simulink model "TrainSimulation_trial"  (R2021a)
settings: Solver=VariableStepAuto  StartTime=0.0  StopTime=10.0  MaxStep=0.01  RelTol=1e-3
values from neighbouring files (symbols this model uses):
  g = 9.8    [TrainSimulation_run.m]
  k = 20    [MassSpringDamper_run.m]    (also in PID_SpringDamper_run.m; PID_block_run.m; TrainSimulation_run.m = 1; TransferFunctionModel_run.m)
  M1 = 1    [TrainSimulation_run.m]
  M2 = 0.5    [TrainSimulation_run.m]
  mu = 0.02    [TrainSimulation_run.m]
settings Model: Creator=shinyh  LastModifiedBy=shinyh

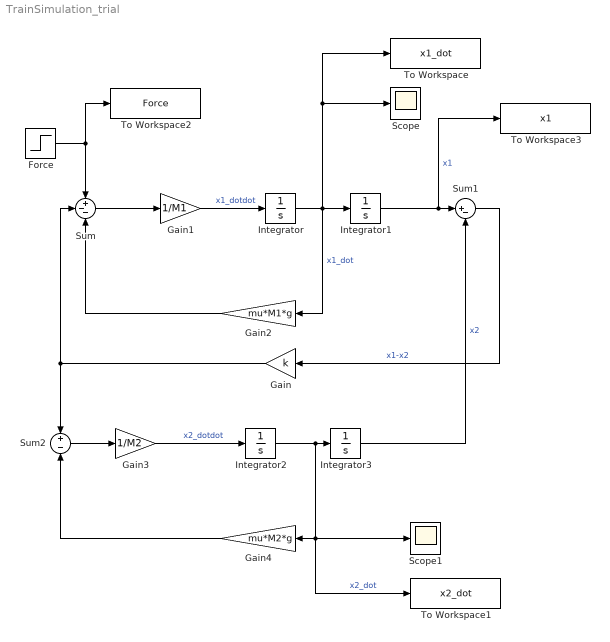
== system TrainSimulation_trial ==
  Force : Step  SampleTime=0
  Gain : Gain  Gain=k
  Gain1 : Gain  Gain=1/M1
  Gain2 : Gain  Gain=mu*M1*g
  Gain3 : Gain  Gain=1/M2
  Gain4 : Gain  Gain=mu*M2*g
  Integrator{,1..3} (4 alike) : Integrator
  Scope : Scope
  Scope1 : Scope
  Sum : Sum  Inputs=+--
  Sum1 : Sum  Inputs=|+-
  Sum2 : Sum  Inputs=+-
  To Workspace : ToWorkspace  VariableName=x1_dot  SaveFormat=Timeseries  SampleTime=-1
  To Workspace1 : ToWorkspace  VariableName=x2_dot  SaveFormat=Timeseries  SampleTime=-1
  To Workspace2 : ToWorkspace  VariableName=Force  SaveFormat=Timeseries  SampleTime=-1
  To Workspace3 : ToWorkspace  VariableName=x1  SaveFormat=Timeseries  SampleTime=-1
  wires:
  Gain1/1 -> Integrator/1  "x1_dotdot"
  Integrator/1 -> To Workspace/1, Scope/1, Gain2/1, Integrator1/1  "x1_dot"
  Integrator1/1 -> To Workspace3/1, Sum1/1  "x1"
  Integrator3/1 -> Sum1/2  "x2"
  Integrator2/1 -> To Workspace1/1, Scope1/1, Gain4/1, Integrator3/1  "x2_dot"
  Gain3/1 -> Integrator2/1  "x2_dotdot"
  Force/1 -> Sum/1, To Workspace2/1
  Sum1/1 -> Gain/1  "x1-x2"
  Sum/1 -> Gain1/1
  Gain2/1 -> Sum/3
  Gain/1 -> Sum/2, Sum2/1
  Sum2/1 -> Gain3/1
  Gain4/1 -> Sum2/2
